simulink model "chapter5_1"  (R2018b)
settings: Solver=VariableStepAuto  StartTime=0.0  StopTime=30  RelTol=1e-3
settings Model: Creator=nharada  LastModifiedBy=nharada

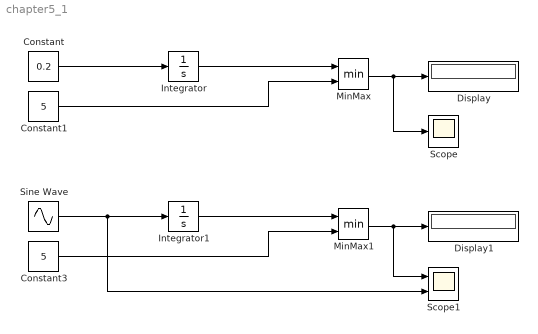
== system chapter5_1 ==
  Constant : Constant  Value=0.2
  Constant1 : Constant  Value=5
  Constant3 : Constant  Value=5
  Display : Display
  Display1 : Display
  Integrator : Integrator
  Integrator1 : Integrator
  MinMax : MinMax  Inputs=2
  MinMax1 : MinMax  Inputs=2
  Scope : Scope
  Scope1 : Scope  NumInputPorts=2
  Sine Wave : Sin  Amplitude=0.2  Bias=0.2  Frequency=pi  SampleTime=0.001
  wires:
  Constant/1 -> Integrator/1
  Constant1/1 -> MinMax/2
  Integrator/1 -> MinMax/1
  MinMax/1 -> Scope/1, Display/1
  MinMax1/1 -> Display1/1, Scope1/1
  Integrator1/1 -> MinMax1/1
  Constant3/1 -> MinMax1/2
  Sine Wave/1 -> Scope1/2, Integrator1/1
